simulink model "Processo_P"  (R2016a)
settings: Solver=VariableStepAuto  StartTime=0.0  StopTime=20  RelTol=1e-3
settings Model: Creator=mende  LastModifiedBy=mende

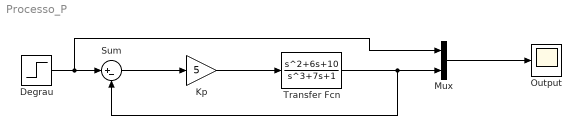
== system Processo_P ==
  Degrau : Step  SampleTime=0
  Kp : Gain  Gain=5
  Mux : Mux  Inputs=2
  Output : Scope
  Sum : Sum  Inputs=|+-
  Transfer Fcn : TransferFcn  Numerator=[1,6,10]  Denominator=[1,0,7,1]
  wires:
  Degrau/1 -> Mux/1, Sum/1
  Transfer Fcn/1 -> Mux/2, Sum/2
  Sum/1 -> Kp/1
  Kp/1 -> Transfer Fcn/1
  Mux/1 -> Output/1
